simulink library "lflib"  (R2016a)
settings: Solver=ode45  StartTime=0.0  StopTime=10.0  RelTol=1e-3
undefined symbols (not defined in the file or in its folder): DiscIntNeverNeededParam, initAngle, initX, initY, Ts
undefined symbols (not defined in the file): S, track_1
libraries: lflib x6, simulink_extras x5
settings Model: Creator=bures  LastModifiedBy=bures
settings DataIOCC: LimitDataPoints=on
settings DebuggingCC: AllowSymbolicDim=off

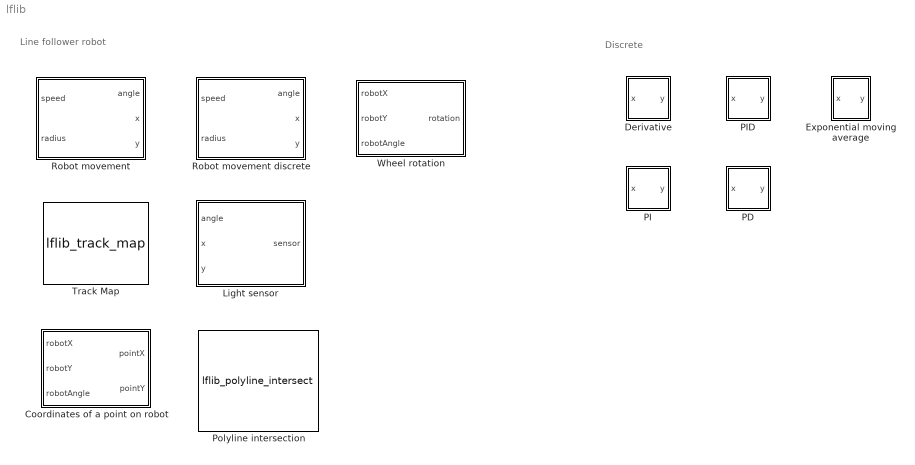
== system lflib ==
  note: Line follower robot
  note: Discrete
  Coordinates of a point on robot : Subsystem  mask{point=S.colorSensor}
  Derivative : Subsystem  mask{Ts=Ts, Fa=0.5}
      mask prompts: Ts "Period"; Fa "Filter coeffiecient"
      mask Display:
      | disp('D');
      | port_label('input', 1, '');
      | port_label('output', 1, '');
  Exponential moving average : Subsystem  mask{alpha=0.5}
      mask Display:
      | disp('EMA');
      | port_label('input', 1, '');
      | port_label('output', 1, '');
  Light sensor : Subsystem  mask{trackCData=track_1, trackSamplesPerM=1000, sensorPos=[150 0]}
      mask prompts: trackCData "Track map"; trackSamplesPerM "Track map samples/m"; sensorPos "Relative sensor position to center (in mm)"
  PD : Subsystem  mask{Kp=1, Kd=0, Smax=100, Smin=-100, Ts=Ts, Dmax=100, Dmin=-100}
      mask prompts: Kp "Proportional gain"; Kd "Derivative gain"; Smax "Saturation - max"; Smin "Saturation - min"; Ts "Period"; Dmax "Derivative Saturation - max"; Dmin "Derivative Saturation - min"
      mask Display:
      | disp('PD');
      | port_label('input', 1, '');
      | port_label('output', 1, '');
  PI : Subsystem  mask{Kp=1, Ki=1, Smax=100, Smin=-100, Ts=Ts, Imax=50, Imin=-50}
      mask prompts: Kp "Proportional gain"; Ki "Integral gain"; Smax "Saturation - max"; Smin "Saturation - min"; Ts "Period"; Imax "Integer Saturation - max"; Imin "Integer Saturation - min"
      mask Display:
      | disp('PI');
      | port_label('input', 1, '');
      | port_label('output', 1, '');
  PID : Subsystem  mask{Kp=1, Ki=0, Kd=0, Smax=inf, Smin=-inf, Ts=Ts, Imax=inf, Imin=-inf, Dmax=inf, Dmin=-inf}
      mask prompts: Kp "Proportional gain"; Ki "Integral gain"; Kd "Derivative gain"; Smax "Saturation - max"; Smin "Saturation - min"; Ts "Period"; Imax "Integer Saturation - max"; Imin "Integer Saturation - min"; Dmax "Derivative Saturation - max"; Dmin "Derivative Saturation - min"
      mask Display:
      | disp('PID');
      | port_label('input', 1, '');
      | port_label('output', 1, '');
  Polyline intersection : M-S-Function  FunctionName=lflib_polyline_intersect  Parameters=line1, line2  mask{line1=[0 0; 1 1], line2=[2 2; 3 3]}
      mask prompts: line1 "Points of polyline 1 (e.g. [0 0; 1 2; 2 0])"; line2 "Points of polyline 2 (e.g. [0 1; 1 0; 0 -1; -1 0; 0 1])"
      mask Display:
      | port_label('input',1,'trX1');
      | port_label('input',2,'trY1');
      | port_label('input',3,'angle1');
      | port_label('input',4,'trX2');
      | port_label('input',5,'trY2');
      | port_label('input',6,'angle2');
      | port_label('output',1,'match');
      | disp('Polyline\nintersection');
  Robot movement : Subsystem  mask{initX=initX, initY=initY, initAngle=initAngle}
      mask prompts: initX "X (in mm)"; initY "Y (in mm)"; initAngle "Angle (in rad)"
  Robot movement discrete : Subsystem  mask{initX=initX, initY=initY, initAngle=initAngle}
      mask prompts: initX "X (in mm)"; initY "Y (in mm)"; initAngle "Angle (in rad)"
  Track Map : M-S-Function  FunctionName=lflib_track_map  Parameters=trackCData, trackSamplesPerM  mask(Track Map){trackCData=track_1, trackSamplesPerM=1000}
      mask prompts: trackCData "Track map"; trackSamplesPerM "Track map samples/m"
      mask Display:
      | disp('Track Map');
      | port_label('input', 1, 'angle');
      | port_label('input', 2, 'x');
      | port_label('input', 3, 'y');
  Wheel rotation : Subsystem  mask{wheelPos=[0 150], initX=initX, initY=initY, initAngle=initAngle}
      mask prompts: wheelPos "Wheel position"; initX "X (in mm)"; initY "Y (in mm)"; initAngle "Angle (in rad)"
      mask DialogControl Container3 Prompt: Initial robot position and orientation

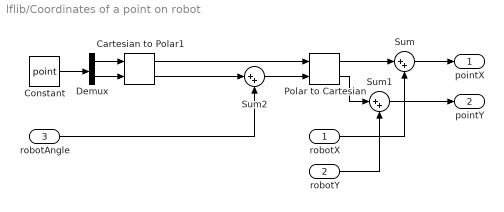
== system lflib/Coordinates of a point on robot ==
  robotX : Inport
  robotY : Inport  Port=2
  robotAngle : Inport  Port=3
  Cartesian to Polar1 : simulink_extras/Transformations/Cartesian to Polar
  Constant : Constant  Value=point
  Demux : Demux  Outputs=2
  Polar to Cartesian : simulink_extras/Transformations/Polar to Cartesian
  Sum : Sum  Inputs=|++
  Sum1 : Sum  Inputs=|++
  Sum2 : Sum  Inputs=|++
  pointX : Outport
  pointY : Outport  Port=2
  wires:
  Constant/1 -> Demux/1
  Demux/2 -> Cartesian to Polar1/2
  Demux/1 -> Cartesian to Polar1/1
  Cartesian to Polar1/2 -> Sum2/1
  robotAngle/1 -> Sum2/2
  Sum2/1 -> Polar to Cartesian/2
  Cartesian to Polar1/1 -> Polar to Cartesian/1
  Polar to Cartesian/1 -> Sum/1
  Sum/1 -> pointX/1
  robotX/1 -> Sum/2
  Polar to Cartesian/2 -> Sum1/1
  robotY/1 -> Sum1/2
  Sum1/1 -> pointY/1

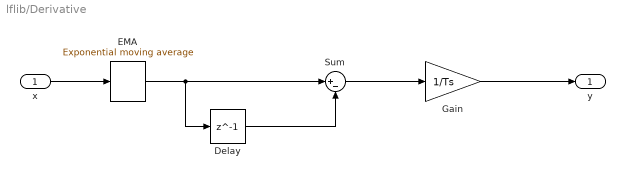
== system lflib/Derivative ==
  x : Inport
  Delay : Delay  DelayLength=1
  EMA : lflib/Exponential moving average  alpha=Fa
  Gain : Gain  Gain=1/Ts  OutDataTypeStr=Inherit: Same as input
  Sum : Sum  Inputs=|+-
  y : Outport
  wires:
  EMA/1 -> Delay/1, Sum/1
  Gain/1 -> y/1
  Sum/1 -> Gain/1
  x/1 -> EMA/1
  Delay/1 -> Sum/2

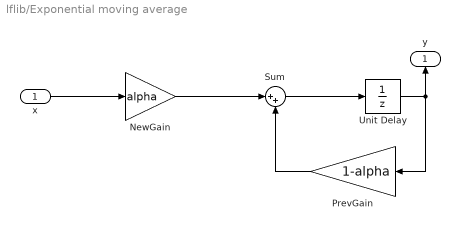
== system lflib/Exponential moving average ==
  x : Inport
  NewGain : Gain  Gain=alpha  OutDataTypeStr=Inherit: Same as input
  PrevGain : Gain  Gain=1-alpha  OutDataTypeStr=Inherit: Same as input
  Sum : Sum  Inputs=|++
  Unit Delay : UnitDelay  SampleTime=-1
  y : Outport
  wires:
  x/1 -> NewGain/1
  Unit Delay/1 -> y/1, PrevGain/1
  Sum/1 -> Unit Delay/1
  PrevGain/1 -> Sum/2
  NewGain/1 -> Sum/1

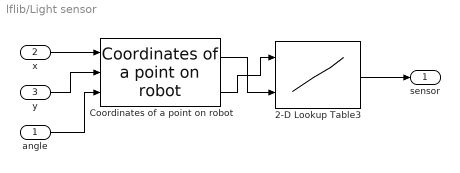
== system lflib/Light sensor ==
  angle : Inport
  x : Inport  Port=2
  y : Inport  Port=3
  2-D Lookup Table3 : Lookup_n-D  BreakpointsForDimension1=[0:1/trackSamplesPerM*1000:(size(trackCData,1)-1)/trackSamplesPerM*1000]  BreakpointsForDimension2=[0:1/trackSamplesPerM*1000:(size(trackCData,2)-1)/trackSamplesPerM*1000]  Table=mean(flipud(double(trackCData)), 3) / 255  ExtrapMethod=Clip  UseLastTableValue=on  RndMeth=Simplest  InputSameDT=on
  Coordinates of a point on robot : lflib/Coordinates of a point on robot  point=sensorPos
  sensor : Outport
  wires:
  2-D Lookup Table3/1 -> sensor/1
  Coordinates of a point on robot/2 -> 2-D Lookup Table3/1
  Coordinates of a point on robot/1 -> 2-D Lookup Table3/2
  angle/1 -> Coordinates of a point on robot/3
  y/1 -> Coordinates of a point on robot/2
  x/1 -> Coordinates of a point on robot/1

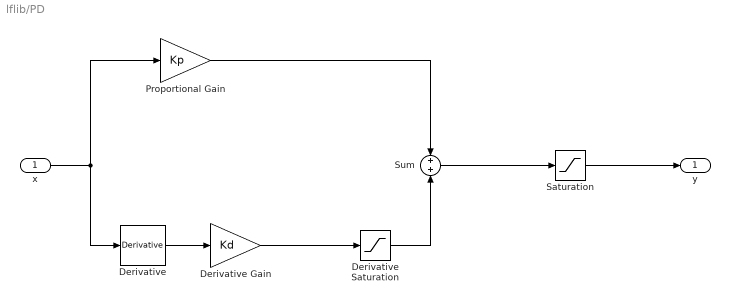
== system lflib/PD ==
  x : Inport
  Derivative : lflib/Derivative  Ts=Ts  Fa=0.5
  Derivative Saturation : Saturate  UpperLimit=Dmax  LowerLimit=Dmin
  Derivative Gain : Gain  DisableCoverage=on  Gain=Kd  OutDataTypeStr=Inherit: Same as input
  Proportional Gain : Gain  DisableCoverage=on  Gain=Kp  OutDataTypeStr=Inherit: Same as input
  Saturation : Saturate  UpperLimit=Smax  LowerLimit=Smin  LinearizeAsGain=off
  Sum : Sum  DisableCoverage=on  Inputs=+|+
  y : Outport
  wires:
  x/1 -> Proportional Gain/1, Derivative/1
  Proportional Gain/1 -> Sum/1
  Saturation/1 -> y/1
  Sum/1 -> Saturation/1
  Derivative/1 -> Derivative Gain/1
  Derivative Gain/1 -> Derivative Saturation/1
  Derivative Saturation/1 -> Sum/2

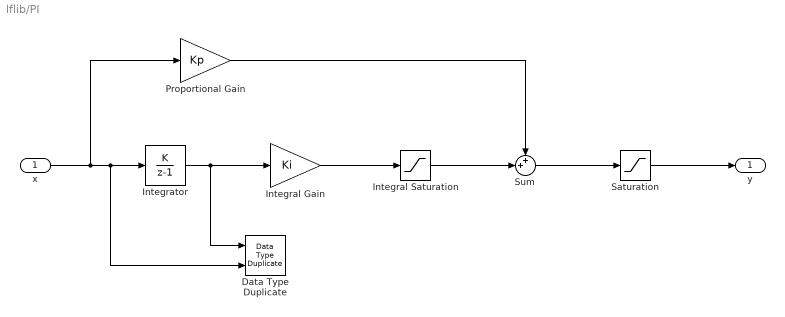
== system lflib/PI ==
  x : Inport
  Data Type Duplicate : DataTypeDuplicate
  Integral Saturation : Saturate  UpperLimit=Imax  LowerLimit=Imin
  Integral Gain : Gain  DisableCoverage=on  Gain=Ki  OutDataTypeStr=Inherit: Same as input
  Integrator : DiscreteIntegrator  DisableCoverage=on  IntegratorMethod=Accumulation: Forward Euler  gainval=Ts  InitialConditionSetting=Compatibility  SampleTime=-1  OutDataTypeStr=Inherit: Inherit via back propagation  ICPrevOutput=DiscIntNeverNeededParam  ICPrevScaledInput=DiscIntNeverNeededParam
  Proportional Gain : Gain  DisableCoverage=on  Gain=Kp  OutDataTypeStr=Inherit: Same as input
  Saturation : Saturate  UpperLimit=Smax  LowerLimit=Smin  LinearizeAsGain=off
  Sum : Sum  DisableCoverage=on  Inputs=++|
  y : Outport
  wires:
  x/1 -> Proportional Gain/1, Integrator/1, Data Type Duplicate/2
  Proportional Gain/1 -> Sum/1
  Saturation/1 -> y/1
  Sum/1 -> Saturation/1
  Integrator/1 -> Integral Gain/1, Data Type Duplicate/1
  Integral Gain/1 -> Integral Saturation/1
  Integral Saturation/1 -> Sum/2

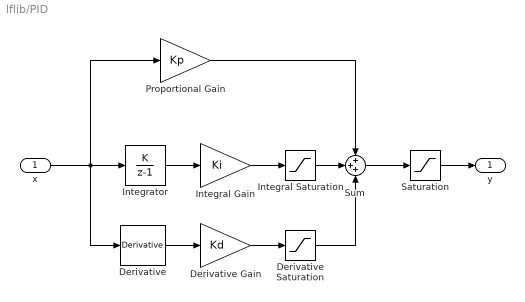
== system lflib/PID ==
  x : Inport
  Derivative : lflib/Derivative  Ts=Ts  Fa=0.5
  Derivative Saturation : Saturate  UpperLimit=Dmax  LowerLimit=Dmin
  Derivative Gain : Gain  DisableCoverage=on  Gain=Kd
  Integral Saturation : Saturate  UpperLimit=Imax  LowerLimit=Imin
  Integral Gain : Gain  DisableCoverage=on  Gain=Ki
  Integrator : DiscreteIntegrator  DisableCoverage=on  IntegratorMethod=Accumulation: Forward Euler  gainval=Ts  InitialConditionSetting=Compatibility  SampleTime=-1  ICPrevOutput=DiscIntNeverNeededParam  ICPrevScaledInput=DiscIntNeverNeededParam
  Proportional Gain : Gain  DisableCoverage=on  Gain=Kp
  Saturation : Saturate  UpperLimit=Smax  LowerLimit=Smin  LinearizeAsGain=off
  Sum : Sum  DisableCoverage=on  Inputs=+++
  y : Outport
  wires:
  Derivative Saturation/1 -> Sum/3
  Derivative Gain/1 -> Derivative Saturation/1
  Derivative/1 -> Derivative Gain/1
  Integral Saturation/1 -> Sum/2
  Integral Gain/1 -> Integral Saturation/1
  Integrator/1 -> Integral Gain/1
  Sum/1 -> Saturation/1
  Saturation/1 -> y/1
  Proportional Gain/1 -> Sum/1
  x/1 -> Integrator/1, Derivative/1, Proportional Gain/1

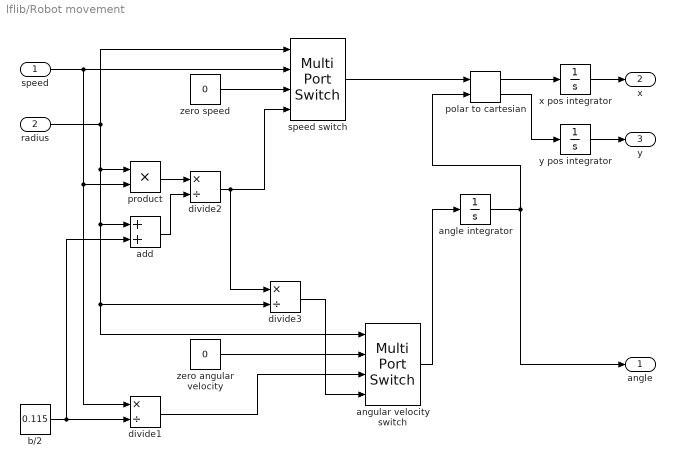
== system lflib/Robot movement ==
  speed : Inport
  radius : Inport  Port=2
  add : Sum
  angle integrator : Integrator  InitialCondition=initAngle
  angular velocity switch : MultiPortSwitch  DataPortOrder=Zero-based contiguous  Inputs=2  DataPortIndices={0,1}  DataPortForDefault=Additional data port  DiagnosticForDefault=None
  b/2 : Constant  Value=0.115
  divide1 : Product  Inputs=*/
  divide2 : Product  Inputs=*/
  divide3 : Product  Inputs=*/
  polar to cartesian : simulink_extras/Transformations/Polar to Cartesian
  product : Product
  speed switch : MultiPortSwitch  DataPortOrder=Zero-based contiguous  Inputs=2  DataPortIndices={0,1}  DataPortForDefault=Additional data port  DiagnosticForDefault=None
  x pos integrator : Integrator  InitialCondition=initX
  y pos integrator : Integrator  InitialCondition=initY
  zero angular velocity : Constant  Value=0
  zero speed : Constant  Value=0
  angle : Outport
  x : Outport  Port=2
  y : Outport  Port=3
  wires:
  divide3/1 -> angular velocity switch/4
  divide2/1 -> speed switch/4, divide3/1
  angular velocity switch/1 -> angle integrator/1
  add/1 -> divide2/2
  product/1 -> divide2/1
  divide1/1 -> angular velocity switch/3
  b/2/1 -> divide1/2, add/2
  zero angular velocity/1 -> angular velocity switch/2
  zero speed/1 -> speed switch/3
  speed switch/1 -> polar to cartesian/1
  speed/1 -> divide1/1, product/2, speed switch/2
  radius/1 -> product/1, add/1, divide3/2, angular velocity switch/1, speed switch/1
  angle integrator/1 -> polar to cartesian/2, angle/1
  y pos integrator/1 -> y/1
  polar to cartesian/2 -> y pos integrator/1
  polar to cartesian/1 -> x pos integrator/1
  x pos integrator/1 -> x/1

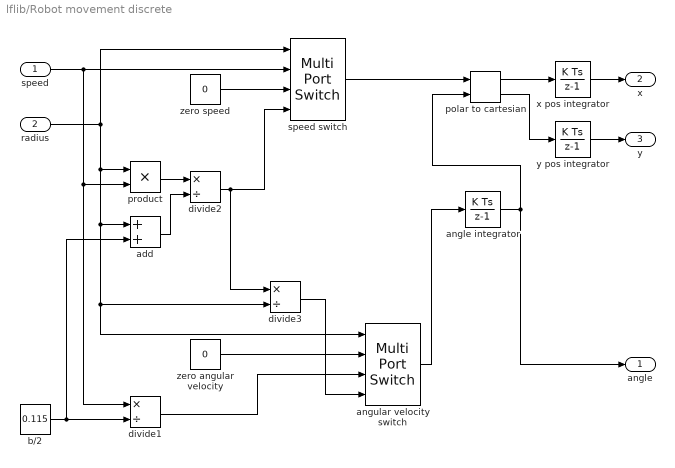
== system lflib/Robot movement discrete ==
  speed : Inport
  radius : Inport  Port=2
  add : Sum
  angle integrator : DiscreteIntegrator  InitialCondition=initAngle  InitialConditionSetting=State (most efficient)  SampleTime=-1  ICPrevOutput=DiscIntNeverNeededParam  ICPrevScaledInput=DiscIntNeverNeededParam
  angular velocity switch : MultiPortSwitch  DataPortOrder=Zero-based contiguous  Inputs=2  DataPortIndices={0,1}  DataPortForDefault=Additional data port  DiagnosticForDefault=None
  b/2 : Constant  Value=0.115
  divide1 : Product  Inputs=*/
  divide2 : Product  Inputs=*/
  divide3 : Product  Inputs=*/
  polar to cartesian : simulink_extras/Transformations/Polar to Cartesian
  product : Product
  speed switch : MultiPortSwitch  DataPortOrder=Zero-based contiguous  Inputs=2  DataPortIndices={0,1}  DataPortForDefault=Additional data port  DiagnosticForDefault=None
  x pos integrator : DiscreteIntegrator  InitialCondition=initX  InitialConditionSetting=State (most efficient)  SampleTime=-1  ICPrevOutput=DiscIntNeverNeededParam  ICPrevScaledInput=DiscIntNeverNeededParam
  y pos integrator : DiscreteIntegrator  InitialCondition=initY  InitialConditionSetting=State (most efficient)  SampleTime=-1  ICPrevOutput=DiscIntNeverNeededParam  ICPrevScaledInput=DiscIntNeverNeededParam
  zero angular velocity : Constant  Value=0
  zero speed : Constant  Value=0
  angle : Outport
  x : Outport  Port=2
  y : Outport  Port=3
  wires:
  x pos integrator/1 -> x/1
  polar to cartesian/1 -> x pos integrator/1
  polar to cartesian/2 -> y pos integrator/1
  y pos integrator/1 -> y/1
  angle integrator/1 -> angle/1, polar to cartesian/2
  radius/1 -> speed switch/1, angular velocity switch/1, divide3/2, add/1, product/1
  speed/1 -> speed switch/2, product/2, divide1/1
  speed switch/1 -> polar to cartesian/1
  zero speed/1 -> speed switch/3
  zero angular velocity/1 -> angular velocity switch/2
  b/2/1 -> add/2, divide1/2
  divide1/1 -> angular velocity switch/3
  product/1 -> divide2/1
  add/1 -> divide2/2
  angular velocity switch/1 -> angle integrator/1
  divide2/1 -> divide3/1, speed switch/4
  divide3/1 -> angular velocity switch/4

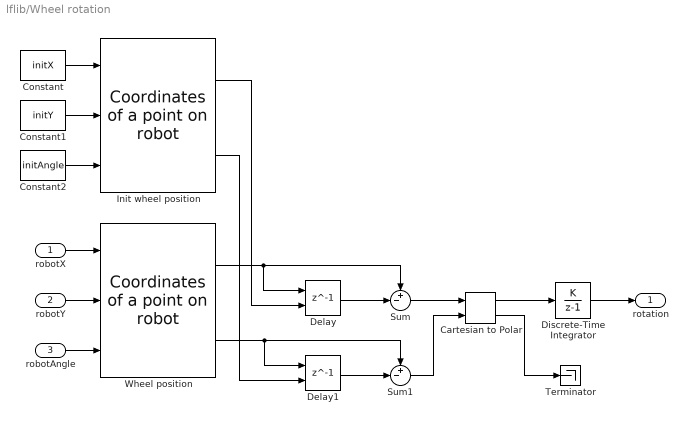
== system lflib/Wheel rotation ==
  robotX : Inport
  robotY : Inport  Port=2
  robotAngle : Inport  Port=3
  Cartesian to Polar : simulink_extras/Transformations/Cartesian to Polar
  Constant : Constant  Value=initX
  Constant1 : Constant  Value=initY
  Constant2 : Constant  Value=initAngle
  Delay : Delay  DelayLength=1  InitialConditionSource=Input port
      settings: InputPortMap=u0,p4
  Delay1 : Delay  DelayLength=1  InitialConditionSource=Input port
      settings: InputPortMap=u0,p4
  Discrete-Time Integrator : DiscreteIntegrator  IntegratorMethod=Accumulation: Forward Euler  InitialConditionSetting=State (most efficient)  SampleTime=-1  ICPrevOutput=DiscIntNeverNeededParam  ICPrevScaledInput=DiscIntNeverNeededParam
  Init wheel position : lflib/Coordinates of a point on robot  point=wheelPos
  Sum : Sum  Inputs=+-|
  Sum1 : Sum  Inputs=+-|
  Terminator : Terminator
  Wheel position : lflib/Coordinates of a point on robot  point=wheelPos
  rotation : Outport
  wires:
  Wheel position/1 -> Sum/1, Delay/1
  Cartesian to Polar/1 -> Discrete-Time Integrator/1
  Delay/1 -> Sum/2
  Wheel position/2 -> Sum1/1, Delay1/1
  Delay1/1 -> Sum1/2
  Sum1/1 -> Cartesian to Polar/2
  Cartesian to Polar/2 -> Terminator/1
  Sum/1 -> Cartesian to Polar/1
  Discrete-Time Integrator/1 -> rotation/1
  robotY/1 -> Wheel position/2
  robotAngle/1 -> Wheel position/3
  robotX/1 -> Wheel position/1
  Constant/1 -> Init wheel position/1
  Constant1/1 -> Init wheel position/2
  Constant2/1 -> Init wheel position/3
  Init wheel position/1 -> Delay/2
  Init wheel position/2 -> Delay1/2
